simulink subsystem "cnt2rad"  (R2022b)
settings: Solver=VariableStepAuto  StartTime=0.0  StopTime=10.0  RelTol=1e-3
undefined symbols (not defined in the file or in its folder): constant
libraries: simulink x1
settings Model: Creator=Alex Zhen  LastModifiedBy=Alex Zhen

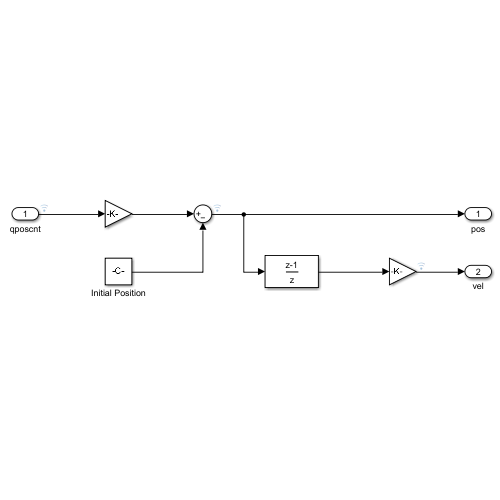
[thumbnail: Simulink's stored preview of the top-level diagram]
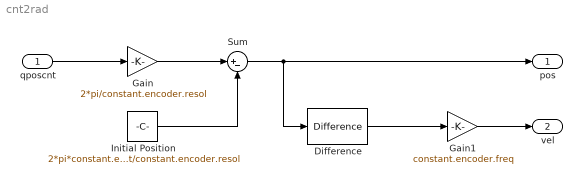
== system cnt2rad ==
  qposcnt : Inport
  Difference : simulink/Discrete/Difference  ICPrevInput=0.0  OutMin=[]  OutMax=[]  OutDataType=fixdt(1, 16)  OutScaling=2^-10  DoSatur=off
  Gain : Gain  Gain=2*pi/constant.encoder.resol
  Gain1 : Gain  Gain=constant.encoder.freq
  Initial Position : Constant  Value=2*pi*constant.encoder.cnt_init/constant.encoder.resol
  Sum : Sum  Inputs=|+-
  pos : Outport
  vel : Outport  Port=2
  wires:
  Sum/1 -> pos/1, Difference/1
  Difference/1 -> Gain1/1
  Gain/1 -> Sum/1
  Gain1/1 -> vel/1
  qposcnt/1 -> Gain/1
  Initial Position/1 -> Sum/2
